simulink model "Leg_Sim_VariableDamping"  (R2020b)
settings: Solver=ode23s  StartTime=0.0  StopTime=1  RelTol=1e-3
values from neighbouring files (symbols this model uses):
  body = Leg_Pars_Body    [Leg_Script_Powered.m]    (also in Leg_Script_Socket_VariableDamping.m; Leg_Script_VariableDamping.m)
  ctrl = Leg_Pars_Ctrl_Powered    [Leg_Script_Powered.m]    (also in Leg_Script_Socket_VariableDamping.m = Leg_Pars_Ctrl_VariableDamping; Leg_Script_VariableDamping.m = Leg_Pars_Ctrl_VariableDamping)
  device = Leg_Pars_Device_Powered    [Leg_Script_Powered.m]    (also in Leg_Script_Socket_VariableDamping.m = Leg_Pars_Device_VariableDamping; Leg_Script_VariableDamping.m = Leg_Pars_Device_VariableDamping)
  FD = [1;1;0;1;1;0;0;1]    [Leg_Script_Powered.m]    (also in Leg_Script_Socket_VariableDamping.m = [1;1;0;1;1;1;1;0;0;1]; Leg_Script_VariableDamping.m)
  human = Leg_Pars_Human(body)    [Leg_Script_Powered.m]    (also in Leg_Script_Socket_VariableDamping.m; Leg_Script_VariableDamping.m)
  intent = [0;1;0]    [Leg_Script_Powered.m]    (also in Leg_Script_Socket_VariableDamping.m; Leg_Script_VariableDamping.m)
  intentv = [1.1;1.1;0.8]    [Leg_Script_Powered.m]    (also in Leg_Script_Socket_VariableDamping.m = [1.1; 1.1; 1.4; 1.4; 1.1; 1.1; 1.4;0.8]; Leg_Script_VariableDamping.m = [1.1; 1.1; 1.4; 1.4; 1.1; 1.1; 1.4;0.8])
  q0 = [0;1;ref.pt_walk ... (first row only)    [Leg_Script_Powered.m]    (also in Leg_Script_Socket_VariableDamping.m; Leg_Script_VariableDamping.m)
  qd0 = [intentv(1)*1.2*intent(1);0;0;0;0;0;0;0]    [Leg_Script_Powered.m]    (also in Leg_Script_Socket_VariableDamping.m = [intentv(1)*1.25*intent(1);0;0;0;0;0;0;0;0;0]; Leg_Script_VariableDamping.m)
  robsim = robotcell2mat(robot)    [Leg_Script_Powered.m]    (also in Leg_Script_Socket_VariableDamping.m; Leg_Script_VariableDamping.m)
  t_intent = [0;1;15]    [Leg_Script_Powered.m]    (also in Leg_Script_Socket_VariableDamping.m = [0;1;35]; Leg_Script_VariableDamping.m = [0;1;35])
  t_intentv = [0;10;15]    [Leg_Script_Powered.m]    (also in Leg_Script_Socket_VariableDamping.m = [0; 9.99; 10; 14.99; 15; 20; 25;35]; Leg_Script_VariableDamping.m = [0; 9.99; 10; 14.99; 15; 20; 25;35])
  u0 = zeros(1,length(robot.gc.body))    [Leg_Script_Powered.m]    (also in Leg_Script_Socket_VariableDamping.m; Leg_Script_VariableDamping.m)
undefined symbols (not defined in the file or in its folder): syst
libraries: simulink x4
(part 2 of 2)

== stateflow chart Leg_Sim_VariableDamping/ctrl/High-level ctrl/Chart ==
  state Walk
    state Swing
      during: tSw = elapsed(sec);
      state SwE
        entry:
        state=5;
      state SwF
        entry:
        state=4;
      (default) -> SwF
      SwF -> SwE [order 1] : [pk<p_5 && wk<-w_0]
    state Stance
      tSt = elapsed(sec);
      tC2PSw = duration(pk<p_3);
      state PSw
        entry:
        state=3;
      state Stand
        state StF
          entry:
          state=1;
        state StE
          entry:
          state=2;
        (default) -> StF
        StF -> StE : [wk<-w_0 && ...
            | duration(pk<p_2)>t_0]
        StE -> StF : [wk>w_1 || ...
            | (wk>w_0 && pk>p_2>t_0)]
      PSw -> Stand [order 2] : [F>F_St ...
          | && pk>p_3 ...
          | && M<M_StX ...
          | || after(t_StX,sec)]
      Stand -> PSw : [M>M_3 && wk>w_0 ...
          | && tC2PSw>t_3]
      (default) -> Stand
    Stance -> Swing : [F<F_Sw ...
        | && pk>p_4]
    SwE -> Stance : [F>F_St ...
        | && pk<p_St ...
        | && after(t_0,sec)]
    SwF -> Stance [order 2] : [F>F_St ...
        | && after(t_0,sec) ...
        | && wk<w_StR && pk<p_StR ...
        | && (pk<p_4 || after(t_StX,sec))]
    PSw -> Swing [order 1] : [F<F_Sw ...
        | || pk>p_4]
    (default) -> Stance
  state InitState
    entry:
    state=0;
  InitState -> Walk : [after(0.1,sec)]
  (default) -> InitState
  data: pk input; wk input; M input; F input; state output; tSw output; tSt output; t_0 constant double =fsm.t_0; p_2 constant double =fsm.p_2; w_1 constant double =fsm.w_1; p_4 constant double =fsm.p_4; p_St constant double =fsm.p_st; w_StR constant double =fsm.w_stR; t_StX constant double =fsm.t_stX; p_StR constant double =fsm.p_stR; M_StX constant double =fsm.M_stX; M_3 constant double =fsm.M_3; t_3 constant double =fsm.t_3; p_3 constant double =fsm.p_3; p_5 constant double =fsm.p_5; w_0 constant double =fsm.w_0; tC2PSw local; F_Sw constant double =fsm.F_Sw; F_St constant double =fsm.F_St

== stateflow chart Leg_Sim_VariableDamping/system/human model/healthy trajectory generator ==
  state Fout = PD2lim(X,Xref,P,D,Flim) [function]
  state Walk
    entry:
    initReStep;
    qcmd(1) = x_heel + l_foot/2;
    qcmd(3) = qs_trunkp_walk;
    during:
    t_ReStep = elapsed(sec);
    t_HeStep = t_ReStep + t_HeStance;
    Ttrunk = PD2lim([q(3) qd(3)],[qref(3) qdref(3)],Ptrr1,Dtrr1,m*5);
    Thip = PD2lim([q(4) qd(4)],[qref(4) qdref(4)],Phip1,Dhip1,m*4);
    state ReStepStart
      during:
      qcmd(4) = interp1x(ts_hip_walkstart, qs_hip_walkstart, t_ReStep/t_ReStep_target);
      state HeSwing
        entry: istate=101;
        F = [0;0];
      state HeStance
        entry: istate=102; initHeStep;
        during:
        t_HeStance = elapsed(sec);
        F = FHeStance;
      Walk.ReStepStart.HeSwing -> Walk.ReStepStart.HeStance : [q(2)<=cos(p_attack)*l_pen_0 ...
          | && after(0.2,sec)]
      (default) -> Walk.ReStepStart.HeSwing
    state ReStepCycle
      during:
      qcmd(4) = interp1x(ts_hip_walk, qs_hip_walk, t_ReStep/t_ReStep_target);
      state DoubleSupport
        entry: istate=110;
        during:
        F = FHeStance;
      state HeSwing
        entry: istate=111;
        F = [0;0];
      state HeStance
        entry: istate=112; initHeStep;
        during:
        t_HeStance = elapsed(sec);
        F = FHeStance;
      Walk.ReStepCycle.HeSwing -> Walk.ReStepCycle.HeStance : [q(2)<=cos(p_attack)*l_pen_0 ...
          | && after(0.2,sec)]
      (default) -> Walk.ReStepCycle.DoubleSupport
      Walk.ReStepCycle.DoubleSupport -> Walk.ReStepCycle.HeSwing : [F_SLIP<0]
    state ReStepStop
      during:
      qcmd(4) = interp1x(ts_hip_stopwalk, qs_hip_stopwalk, t_ReStep/t_ReStep_target);
      state DoubleSupport
        entry: istate=120;
        during:
        F = FHeStance;
      state HeSwing
        entry: istate=121;
        F = [0;0];
      state HeStanceStop
        entry: istate=122; initHeStep;
        during:
        t_HeStance = elapsed(sec);
        F = FHeStance;
      Walk.ReStepStop.HeSwing -> HeStanceStop : [q(2)<=cos(p_attack)*l_pen_0 ...
          | && after(0.2,sec)]
      (default) -> Walk.ReStepStop.DoubleSupport
      Walk.ReStepStop.DoubleSupport -> Walk.ReStepStop.HeSwing : [F_SLIP<0]
  state Init
    entry: qcmd = q0(1:4);
  state Stand
    entry: istate = 0;
    disp(['Stand: t = ' sprintf('%.3f',t) ' s.'])
    t_delay=0.2;
    qcmd = [x_heel+l_foot/2;
    qs_trunky_rest;
    qs_trunkp_rest;
    qs_hip_rest];
    during:
    Ttrunk = PD2lim([q(3) qd(3)],[qref(3) qdref(3)],Ptrr0,Dtrr0,m*2.5);
    Thip = PD2lim([q(4) qd(4)],[qref(4) qdref(4)],Phip0,Dhip0,m*2);
    F = [-50*qd(1);
    m*g*0.5];
  Init -> Walk.ReStepCycle.HeSwing [order 2] : [intent==1]
      | {v_HeAmb_target = intentv;}
  (default) -> Init
  Init -> Stand [order 1] : [intent==0]
  Stand -> ReStepStart : [intent==1]
      | {v_HeAmb_target = intentv;}
  Walk.ReStepStart.HeStance -> (junction 379) : [t_ReStep> t_ReStep_target*0.9 && after(0.2,sec) && fy_heel>1]
  (junction 379) -> ReStepCycle
  (junction 380) -> ReStepCycle [order 1] : [intent==1]
  Walk.ReStepCycle.HeStance -> (junction 380) : [t_ReStep> t_ReStep_target*0.9 && after(0.2,sec) && fy_heel>1]
  HeStanceStop -> Stand : [t_ReStep> t_ReStep_target*0.9 && (qcmd(1)-q(1))<0.01 && after (0.2,sec) && fy_heel>1]
  (junction 380) -> ReStepStop [order 2]
  data: Vq function_output; X function_input; V function_input; Xq function_input; X function_input double size=[1 2]; Xref function_input double size=[1 2]; P function_input double size=1; D function_input double size=1; Fout function_output size=1; Flim function_input double size=1; Fout function_output; qcmd output size=4; fy_heel input; x_heel input; intent input; t_delay output =0.2; ts_hip_walk constant double size=size(ref.th_walk) =ref.th_walk; qs_hip_walk constant double size=size(ref.ph_walk) =ref.ph_walk; qs_trunky_rest constant double =1; qs_trunkp_rest constant double =ref.pt_stand; qs_hip_rest constant double =ref.ph_stand; qs_hip_walkstart constant double size=size(ref.ph_walkstart) =ref.ph_walkstart; ts_hip_walkstart constant double size=size(ref.th_walkstart) =ref.th_walkstart; q0 constant double size=size(q0) =q0; qs_trunkp_walk constant double =ref.pt_walk; istate output =0; l_foot constant double =bdy.x_ball-bdy.x_heel; ts_hip_stopwalk constant double size=size(ref.th_walkstop) =ref.th_walkstop; qs_hip_stopwalk constant double size=size(ref.ph_walkstop) =ref.ph_walkstop; x_Step_est local double =x_step_0; t_ReStep_target local =x_step_0/intentv(1); intentv input; Dtrr1 constant double =imp.Dt_walk; m constant double =bdy.m; q input; qd input; Ptrr1 constant double =imp.Pt_walk; p_attack constant double =SLIP.p_attack; F output; Ttrunk output; Thip output; v_Amb output =intentv(1); Kthrust output =Kthrust_0; F_SLIP local; t_HeStance local =0; Dhip0 constant double =imp.Dh_stand; Phip0 constant double =imp.Ph_stand; Ptrr0 constant double =imp.Pt_stand; g constant double =-rob.gravity(2); Dhip1 constant double =imp.Dh_walk; Phip1 constant double =imp.Ph_walk; q1_Re local =0; m_trunk constant double =bdy.m_trunk; d_slip local; k_slip local; x_pen_0 output; qref input size=4; qdref input size=4; t_HeStep_target local =x_step_0/intentv(1); v_HeAmb_target local =intentv(1); v_HeAmb_target_prev local =intentv(1); v_ReAmb_target local =intentv(1); t_ReStep output =1; v_ReAmb local =intentv(1); v_HeAmb local =intentv(1); q1_He local =0; l_pen_0 local =SLIP.l_rest; Fy_SLIPsupport_max local =0; Dtrr0 constant double =imp.Dt_stand; t input; t_HeStep local =1
  function initReStep:
    | function initReStep
    | disp(['Walk, step residual leg: t = ' sprintf('%.3f',t) ' s.'])
    | % initialize walking parameters
    | % updates
    | q1D = q(1) - q1_Re;
    | q1_Re = q(1);
    | v_ReAmb = q1D/t_ReStep;
    | v_Amb = v_ReAmb;
    | % update time-based targets
    | v_ReAmb_target = intentv;
    | if istate==112
    |     x_Step_est = q1D;
    | end
    | t_ReStep_target = x_Step_est / v_ReAmb_target;
    | t_delay=0.1*t_ReStep_target;
  function Vq = interp1x(X,V,Xq):
    | function Vq = interp1x(X,V,Xq)
    | % interp1x is identical to interp1 except that lower and upper
    | % extrapolation attempts don't result in NaN but in begin and end values,
    | % respectively.
    | Vq = interp1(X,V,max(min(Xq,max(X)),min(X)));
  function initHeStep:
    | function initHeStep
    | disp(['Walk, step intact leg: t = ' sprintf('%.3f',t) ' s.'])
    | % (1) update walking speed
    | q1D = q(1) - q1_He;
    | q1_He = q(1);
    | v_HeAmb = q1D/t_HeStep;
    | v_Amb = v_HeAmb;
    | % set target velocity
    | v_HeAmb_target_prev = v_HeAmb_target; % save previous target
    | v_HeAmb_target = v_ReAmb_target; % new target (= residual leg target velocity)
    | % (2) if not in starting walk stance state, update thrust force
    | if istate ~=102
    |     % use target based on averaging current and previous (simple FIR filter)
    |     v_HeAmb_target_ref = (v_HeAmb_target_prev + v_ReAmb_target)/2;
    |     % calc difference in kinetic energy
    |     ED = m/2*(v_HeAmb_target_ref^2 - v_HeAmb^2);
    |     % adjust thrust force
    |     Kthrust = Kthrust + ED/(x_Step_est*0.5*v_HeAmb_target_ref^2);
    | end
    | % (3)initialize SLIP parameters
    | % calcs
    | t_HeStep_target = x_Step_est / v_HeAmb_target;
    | zeta = 0.2; % damping ratio of SLIP model
    | k_slip = m_trunk*(2*pi/(t_HeStep_target*0.5/2)/sqrt(1-zeta^2))^2;
    | d_slip = zeta*2*sqrt(k_slip*m_trunk); % [Ns/m] damping
    | x_pen_0 = q(1)+sin(p_attack)*l_pen_0;
    | F_SLIP = 0;
    | % SLIP Support
    | Fy_SLIPsupport_max = 0.1*k_slip*(1.1 - v_ReAmb_target);
  function Fout = FHeStance:
    | function Fout = FHeStance
    | % SLIP calculations
    | x_pen = q(1) - x_pen_0;
    | l_pen = sqrt(x_pen^2+q(2)^2);
    | l_pend = (x_pen*qd(1) + q(2)*qd(2))/l_pen;
    | Fk = -k_slip*(l_pen - l_pen_0);
    | Fd = -d_slip*l_pend;
    | F_SLIP = Fk + Fd;
    | Fout = [F_SLIP*x_pen/l_pen;F_SLIP*q(2)/l_pen];
    | 
    | % Add horizontal and vertical support force
    | Fx_support = 0;
    | Fy_support = 0;
    | p_pen = asin(x_pen/l_pen);
    | % Add vertical vertical support force for slow speeds
    | if Fy_SLIPsupport_max>0
    |     p_pen = asin(x_pen/l_pen);
    |     if abs(p_pen)<p_attack
    |         %      Fout(2) = Fout(2) + Fy_SLIPsupport_max/2*(1+cos(p_pen*pi/p_attack));
    |         Fy_support = Fy_SLIPsupport_max*(cos(p_pen*pi/2/p_attack));
    |     end
    | end
    | if istate == 122 % different support for terminating state
    |     % Add horizontal thrust force (without speed change compensation)
    |     Fx_support =  -m*v_HeAmb/(sin(p_attack)*l_pen_0)*qd(1);
    |     % Add addition vertical support for stopping
    |     timefact = max(min(1,1-(t_HeStance-t_HeStep_target/4)/(t_HeStep_target/4)),0);
    |     if abs(p_pen)<p_attack
    |         Fy_support = Fy_support + timefact*0.04*k_slip*(cos(p_pen*pi/2/p_attack));
    |     end
    |     
    | else
    |     % Add horizontal thrust force
    |     Fx_support = v_HeAmb_target^2*Kthrust + ...
    |         0.5*m/2*(v_HeAmb_target^2-v_HeAmb_target_prev^2)/(sin(p_attack)*l_pen_0*2);
    | end
    | 
    | % sum together
    | Fout = Fout + [Fx_support;Fy_support];

== matlab function Leg_Sim_VariableDamping/system/HDgc/HD ==
  data: vJ input; Xup input; v input; Xa input; qdd_id input; tau_fd input; f_ext input; model parameter; fd parameter; qdd_fd output; tau_id output
function [qdd_fd,tau_id] = HD(vJ, Xup, v, Xa, qdd_id, tau_fd, f_ext, model, fd)

% HD  Articulated-Body Hybrid Dynamics Algorithm
% [qdd_fd,tau_id] = HD(vJ, Xup, v, Xa, qdd_id, tau_fd, f_ext, model, fd)
% calculates the hybrid dynamics of a kinematic tree using the articulated-body algorithm. 

% extract statics
ND = model.ND; % 3 = planar, 6 = spatial (note: spatial is not operational in the present implementation)
NB = model.NB;
NB_fd = model.NB_fd;
NB_id = model.NB_id;
S = model.S;
fd_i = model.fd_i;
id_i = model.id_i;
a_grav = model.a_grav;

% pre-allocating variables
c = zeros(ND,NB);
IA = zeros(ND,ND,NB);
pA = zeros(ND,NB);
U = zeros(ND,NB);
d = zeros(NB,1);
u = zeros(NB,1);
a = zeros(ND,NB);

% calculate c (= Sdot*qdot)
for i = 1:NB
    if model.parent(i) ~= 0
        c(:,i) = crm(v(:,i)) * vJ(:,i);
    end
    if fd(i) == 0
        c(:,i) = c(:,i) + S(:,i) * qdd_id(id_i(i));
    end
end

% rigid-body inertia and bias force in body coordinates
for i = 1:NB
    IA(:,:,i) = model.I(:,:,i);
    pA(:,i) = crf(v(:,i)) * model.I(:,:,i) * v(:,i);
    if numel(f_ext)>1 % apply external forces
        pA(:,i) = pA(:,i) - Xa(:,:,i)' \ f_ext(:,i);
    end
end

% forces and inertia [recursive]
for i = NB:-1:1
    if fd(i) == 0
        if model.parent(i) ~= 0
            Ia = IA(:,:,i);
            pa = pA(:,i) + IA(:,:,i)*c(:,i);
            IA(:,:,model.parent(i)) = IA(:,:,model.parent(i)) + Xup(:,:,i)' * Ia * Xup(:,:,i);
            pA(:,model.parent(i)) = pA(:,model.parent(i)) + Xup(:,:,i)' * pa;
        end
    else
        U(:,i) = IA(:,:,i) * S(:,i);
        d(i) = S(:,i)' * U(:,i);
        u(i) = tau_fd(fd_i(i)) - S(:,i)'*pA(:,i);
        if model.parent(i) ~= 0
            Ia = IA(:,:,i) - U(:,i)/d(i)*U(:,i)';
            pa = pA(:,i) + Ia*c(:,i) + U(:,i) * u(i)/d(i);
            IA(:,:,model.parent(i)) = IA(:,:,model.parent(i)) + Xup(:,:,i)' * Ia * Xup(:,:,i);
            pA(:,model.parent(i)) = pA(:,model.parent(i)) + Xup(:,:,i)' * pa;
        end
    end
end

% joint acceleration and torque (in joint space) [recursive]
qdd_fd = zeros(NB_fd,1); 
tau_id = zeros(NB_id,1);

for i = 1:NB
    if model.parent(i) == 0
        a(:,i) = Xup(:,:,i) * -a_grav + c(:,i);
    else
        a(:,i) = Xup(:,:,i) * a(:,model.parent(i)) + c(:,i);
    end
    if fd(i) == 0
        tau_id(id_i(i)) = S(:,i)'*(IA(:,:,i)*a(:,i) + pA(:,i));
    else
        qdd_fd(fd_i(i)) = (u(i) - U(:,i)'*a(:,i))/d(i);
        a(:,i) = a(:,i) + S(:,i)*qdd_fd(fd_i(i));
    end
end

function  vcross = crm( v )

% crm  spatial/planar cross-product operator (motion).
% crm(v)  calculates the 6x6 (or 3x3) matrix such that the expression
% crm(v)*m is the cross product of the motion vectors v and m.  If
% length(v)==6 then it is taken to be a spatial vector, and the return
% value is a 6x6 matrix.  Otherwise, v is taken to be a planar vector, and
% the return value is 3x3.

if length(v) == 6
    
    vcross = [  0    -v(3)  v(2)   0     0     0    ;
        v(3)  0    -v(1)   0     0     0    ;
        -v(2)  v(1)  0      0     0     0    ;
        0    -v(6)  v(5)   0    -v(3)  v(2) ;
        v(6)  0    -v(4)   v(3)  0    -v(1) ;
        -v(5)  v(4)  0     -v(2)  v(1)  0 ];
    
else
    
    vcross = [  0     0     0    ;
        v(3)  0    -v(1) ;
        -v(2)  v(1)  0 ];
end

function  vcross = crf( v )

% crf  spatial/planar cross-product operator (force).
% crf(v)  calculates the 6x6 (or 3x3) matrix such that the expression
% crf(v)*f is the cross product of the motion vector v with the force
% vector f.  If length(v)==6 then it is taken to be a spatial vector, and
% the return value is a 6x6 matrix.  Otherwise, v is taken to be a planar
% vector, and the return value is 3x3.

vcross = -crm(v)';

== matlab function Leg_Sim_VariableDamping/system/HDgc/transcalc ==
  data: q input; qd input; vJ output; model parameter; Xup output; v output; Xa output
function [vJ, Xup, v, Xa] = transcalc( q, qd, model)
% [vJ, Xup, v, Xa] = transcalc( q, qd, model)
% calculates vectors of
% joint velocities vJ;
% body transformations Xup (Xjoint + Xtree);
% body velocities v (w.r.t. global);
% body transformations Xa (w.r.t. global);

% extract statics
ND = model.ND; % 3 = planar, 6 = spatial (note: spatial is not operational in the present implementation)
NB = model.NB;
S = model.S;

% pre-allocating variables
Xup = zeros(ND,ND,NB);
vJ = zeros(ND,NB);

% calculate body transformations and joint velocity
for i = 1:NB
    XJ = jcalc( model.jtype(i,:), q(i) );
    vJ(:,i) = S(:,i)*qd(i);
    Xup(:,:,i) = XJ * model.Xtree(:,:,i);
end

% calculate body velocity and absolute transformations
v = vJ; % 
Xa = Xup; % xform abs coords (pre-allocate)
for i = 1:NB
    if model.parent(i) ~= 0
        v(:,i) = Xup(:,:,i)*v(:,model.parent(i)) + vJ(:,i);
        Xa(:,:,i) = Xup(:,:,i) * Xa(:,:,model.parent(i));
    end
end

function  Xj = jcalc( jtyp, q )

% jcalc  joint transform matrix.
% Xj = jcalc(type,q)  returns the joint transform matrix
% for a joint of the given type.  jtyp can be either a string or a
% structure containing a string-valued field called 'code'.  Either way,
% the string contains the joint type code.  For joints that take
% parameters (e.g. helical), jtyp must be a structure, and it must contain
% a field called 'pars', which in turn is a structure containing one or
% more parameters.  (For a helical joint, pars contains a parameter called
% 'pitch'.)  q is the joint's position variable.

if ischar( jtyp )
    code = jtyp;
else
    code = jtyp.code;
end

switch code % spatial configurations disabled
%     case 'Rx'				% revolute X axis
%         Xj = rotx(q);
%     case 'Ry'				% revolute Y axis
%         Xj = roty(q);
%     case 'Rz'       		% revolute Z axis
%         Xj = rotz(q);
%     case 'Px'				% prismatic X axis
%         Xj = xlt([q 0 0]);
%     case 'Py'				% prismatic Y axis
%         Xj = xlt([0 q 0]);
%     case 'Pz'   			% prismatic Z axis
%         Xj = xlt([0 0 q]);
%     case 'Hz'				% helical (Z axis)
%         Xj = rotz(q) * xlt([0 0 q*jtyp.pars.pitch]);
    case 'rz'				% planar revolute
        Xj = plnr( q, [0 0] );
    case 'px'				% planar prismatic X axis
        Xj = plnr( 0, [q 0] );
    case 'py'				% planar prismatic Y axis
        Xj = plnr( 0, [0 q] );
    otherwise
        error( 'unrecognised joint code ''%s''', code );
end

function  [o1,o2] = plnr( i1, i2 )

% plnr  compose/decompose planar-vector coordinate transform.
% X=plnr(theta,r) and [theta,r]=plnr(X)  compose a planar-vector coordinate
% transform X from its component parts theta and r, and decompose it into
% those parts, respectively.  theta is a scalar and r is a 2D vector.  r is
% returned as a column vector, but it can be supplied as a row or column
% vector.  X is the transform from A to B coordinates, in which frame B is
% located at point r (expressed in A coordinates) and is rotated by an
% angle theta (radians) relative to frame A.  If two arguments are supplied
% then they are assumed to be theta and r, otherwise X.

if nargin == 2				% theta,r --> X
    
    c = cos(i1);
    s = sin(i1);
    
    o1 = [        1          0  0 ;
        s*i2(1)-c*i2(2)   c  s ;
        c*i2(1)+s*i2(2)  -s  c ];
    
else					% X --> theta,r
    
    c = i1(2,2);
    s = i1(2,3);
    
    o1 = atan2(s,c);
    o2 = [ s*i1(2,1)+c*i1(3,1); s*i1(3,1)-c*i1(2,1) ];
    
end

== matlab function Leg_Sim_VariableDamping/system/HDgc/gcPosVel ==
  data: v input; Xa input; xc output; xcd output; model parameter
function [xc,xcd] = gcPosVel( v, Xa, model )

% gcPosVel  calculate positions and velocities of contact points
% [xc,xcd] = gcPosVel(v, Xa,model) calculates 2xn or 3xn matrices,
% depending on whether the model is planar or spatial,
% containing the position xc and linear velocity xcd of every point
% specified in model.gc.point (n==length(model.gc.point)).
% All are expressed in base (i.e., absolute) coordinates.  The
% data for model.gc.point(i) appears in column i.

% pre-allocating variables
ND = model.ND; % 3 = planar, 6 = spatial
xc = zeros(ND/3+1,length(model.gc.body));
xcd = xc;

% calculate contact point position and velocities
for i = 1:model.NB %unique(model.gc.body);
    if any(i==model.gc.body)
    X = inv(Xa(:,:,i));			% xform body i -> abs coords
    va = X * v(:,i);			% body i vel in abs coords
    iset = model.gc.body == i;		% set of points assoc with body i
    pt = Xpt( X, model.gc.point(:,iset), ND );	% xform points to abs coords
    vpt = Vpt( va, pt, ND );			% linear velocities of points
    xc(:,iset) = pt;		% insert into correct columns
    xcd(:,iset) = vpt;
    end
end

function  xp = Xpt( X, p, ND )

% Xpt  apply Plucker/planar coordinate transform to 2D/3D points
% xp=Xpt(X,p,ND)  applies the coordinate transform X to the points in p,
% returning the new coordinates in xp.  If ND==6 then X is taken to be a
% 6x6 matrix and a Plucker coordinate transform, and p is expected to be a
% 3xn matrix of 3D points.  Otherwise, X is assumed to be a planar
% coordinate transform and p a 2xn array of 2D points.

if ND==6			% 3D points
  E = X(1:3,1:3);
  r = -skew(E'*X(4:6,1:3));
else					% 2D points
  E = X(2:3,2:3);
  r = [ X(2,3)*X(2,1)+X(3,3)*X(3,1); X(2,3)*X(3,1)-X(3,3)*X(2,1) ];
end

xp = E * (p - repmat(r(1:2),1,size(p,2)));

function  vp = Vpt( v, p, ND )

% Vpt  spatial/planar velocities --> velocities at points
% vp=Vpt(v,p,ND)  calculates the linear velocities vp at one or more points p
% due to one or more spatial/planar velocities v.  In 3D, v is either 6x1
% or 6xn, and p and vp are 3xn.  In 2D, v is either 3x1 or 3xn, and p and
% vp are 2xn.  If v is just a single spatial/planar vector then it applies
% to every point in p; otherwise, vp(:,i) is calculated from v(:,i) and
% p(:,i).

if size(v,2)==1 && size(p,2)>1
    v_op = repmat(v,1,size(p,2));
else
    v_op = v;
end

if ND==6				% 3D points and velocities
    vp = v_op(4:6,:) + cross(v_op(1:3,:),p,1);
else					% 2D points and velocities
    vp = v_op(2:3,:) + [ -v_op(1,:).*p(2,:); v_op(1,:).*p(1,:) ];
end

% function  out = skew( in )
% 
% % skew  convert 3D vector <--> 3x3 skew-symmetric matrix
% % S=skew(v) and v=skew(A) calculate the 3x3 skew-symmetric matrix S
% % corresponding to the given 3D vector v, and the 3D vector corresponding
% % to the skew-symmetric component of the given arbitrary 3x3 matrix A.  For
% % vectors a and b, skew(a)*b is the cross product of a and b.  If the
% % argument is a 3x3 matrix then it is assumed to be A, otherwise it is
% % assumed to be v.  skew(A) produces a column-vector result, but skew(v)
% % will accept a row or column vector argument.
% 
% if all(size(in)==[3 3])			% do v = skew(A)
%   out = 0.5 * [ in(3,2) - in(2,3);
% 		in(1,3) - in(3,1);
% 		in(2,1) - in(1,2) ];
% else					% do S = skew(v)
%   out = [  0,    -in(3),  in(2);
% 	   in(3),  0,    -in(1);
% 	  -in(2),  in(1),  0 ];
% end

== matlab function Leg_Sim_VariableDamping/system/HDgc/gcontact ==
  data: f output size=[2 length(model.gc.body)]; fcone output size=[1 length(model.gc.body)]; ud output size=[1 length(model.gc.body)]; p input size=[2 length(model.gc.body)]; pd input size=[2 length(model.gc.body)]; u input size=[1 length(model.gc.body)]; model parameter
function [f, fcone, ud] = gcontact( p, pd, u, model)

% gcontact  calculate 2D/3D ground reaction forces due to compliant contact
% [f, fcone, ud] = gcontact(p, pd, u, model)  calculates the ground-reaction
% forces acting on a set of points due to contact with a compliant ground
% plane.  In 3D, the x-y plane is the ground plane, and z is up.  In 2D,
% the x axis is the ground plane and y is up.  
% model.gc.K, model.gc.D and model.gc.mu are scalars
% giving the stiffness, damping and friction coefficients of the ground
% plane.  p and pd are (nD)x(np) matrices giving the positions and
% velocities of a set of np points in nD-dimensional space (nD=2 or 3).
% gcontact uses the size of p to determine whether it is working in 2D or
% 3D space.  u is an (nD-1)x(np) matrix containing the tangential
% deformation state variables used to implement the friction model.  f is
% an (nD)x(np) matrix of calculated ground-reaction forces.  If f(nD,i)==0
% then point i is not in contact; and if f(nD,i)>0 then point i is in
% contact.  ud is the time derivative of u; and fcone is a 1x(np) matrix
% indicating the stick/slip status of each point.  If fcone(i)<=1 then
% point i is sticking.  This can happen only if point i is in contact.

% Implementation note:  This function implements the nonlinear
% spring-damper model described in Azad & Featherstone "Modelling the
% Contact Between a Rolling Sphere and a Compliant Ground Plane", ACRA
% 2010, Brisbane, Australia, Dec. 1-3.  However, the implementation here is
% for points rather than spheres.

% extract relevant parameters from model structure
K = model.gc.K;
D = model.gc.D;
mu = model.gc.mu;

% Normal force calculation
z = p(end,:);
zd = pd(end,:);
zr = sqrt(max(0,-z));

fn = zr .* ((-K)*z - D*zd);

if mu == 0			% special case: modelling frictionless
  f = max( 0, fn );		% contact, so return the normal force now
  return
end

% Algorithm for full normal+tangent force calculation: (1) set all output
% variables to their correct no-contact values; (2) correct all the values
% that are wrong because their respective points are in contact.  Step (2)
% is subdivided into (2a) calculate correct values for sticking; (2b)
% adjust the values for those points that are found to be slipping; (2c)
% make the corrections to the output variables.

% Step 1: set output variables to correct no-contact values

[nd,np] = size(p);
f = zeros(nd,np);
ud = (-K/D) * u;
fcone = repmat(2,1,np);			% 2 is just an arbitrary value > 1

in_ctact = fn > 0;

% Step 2: correct all those values that are wrong because their respective
% points are in contact.  Note: variables with names ending in c have one
% column for each point that is in contact.
if any(in_ctact)

  % Step 2a: calculate correct values for sticking

  fnc = fn(in_ctact);
  udc = pd(1:end-1,in_ctact);

  zrc = repmat(zr(in_ctact),nd-1,1);
  Kc = K * zrc;
  Dc = D * zrc;
  fKc = Kc .* u(:,in_ctact);

  ftc = -fKc - Dc .* udc;		% correct tangent force for sticking

  % now test for slipping

  fslip = mu * fnc;
  if nd == 3				% 3D contact
    ftcmag = sqrt(sum(ftc.^2,1));
  else					% 2D contact
    ftcmag = abs(ftc);
  end
  fconec = ftcmag ./ fslip;
  slipping = fconec > 1;

  % Step 2b: adjust values for those points that are found to be slipping

  if any(slipping)
    attenuator = repmat(fconec(slipping),nd-1,1);
    fts = ftc(:,slipping) ./ attenuator;
    ftc(:,slipping) = fts;
    udc(:,slipping) = -(fts + fKc(:,slipping)) ./ Dc(:,slipping);
  end

  % Step 2c: apply the corrections to the output variables
  
  f(:,in_ctact) = [ftc;fnc];
  ud(:,in_ctact) = udc;
  fcone(in_ctact) = min(2,fconec);

end

== matlab function Leg_Sim_VariableDamping/system/HDgc/Fpt ==
  data: p input; fp input; f_ext output size=[3 model.NB]; model parameter
function  f_ext = Fpt( p, fp , model)

% Fpt  forces at points --> spatial/planar forces
% f_ext = Fpt(p, fp, model)  converts one or more linear forces fp acting
% at one or more points p to their equivalent spatial or planar forces.
% In 3D, fp and p are 3xn arrays and f is 6xn.  In 2D, fp and p are 2xn and
% f is 3xn.  In both cases, f(:,i) is the equivalent of fp(:,i) acting at
% p(:,i).

% extract statics
ND = model.ND; % 3 = planar, 6 = spatial
NB = model.NB;
b = model.gc.body; % b(i) == body number of point i

if ND == 6		% 3D forces at 3D points
  f_gc = [ cross(p,fp,1); fp ];
else					% 2D forces at 2D points
  f_gc = [ p(1,:).*fp(2,:) - p(2,:).*fp(1,:); fp ];
end

% array sizes
f_gc = reshape( f_gc, ND, length(b) );
f_ext = zeros(ND,NB); % pre-allocate
% for each body i that is mentioned at least once, calculate the sum of
% all forces acting on that body
for i = 1:NB
    if any(i==b)
    f_ext(:,i) = sum( f_gc(:,b==i), 2 );
    end
end

== matlab function Leg_Sim_VariableDamping/system/HDgc/Pgc ==
  data: PgcStick output; f input size=[2 length(model.gc.body)]; ud input; pd input; PgcSlip output
function [PgcStick, PgcSlip] = Pgc( f, ud, pd )
% Calculates power loss from sticking (damping) and slipping (sliding).
PgcStick = f(1,:)*ud' + f(2,:)*pd(2,:)';
PgcSlip = f(1,:)*(pd(1,:)-ud)';

== matlab function Leg_Sim_VariableDamping/ctrl/Mid-level ctrl/Mid Ctrl ==
  data: pk input; state input; mid parameter; cmd_m output
function cmd_m = cmds(pk,state,mid)
% pk: knee angle [rad] (old: q)
% state: state {1...5} (integer)
% mid: parameter structure mid-level ctrl

% if nonsense state (e.g. fail, init), make control law act according to:
if all(state~=1:5)
    state = 1;
end

cmd_m = 0;
% % pkd2 = wk_fmed*abs(wk_fmed);
if state==1
    cmd_m = mid.c_StF;
elseif state==2 % velocity max 2 rad/s, torque max 2*75 Nm
    cmd_m = mid.c_StE;
elseif state==3
    cmd_m = mid.c_PSw;
elseif state==4
    cmd_m = mid.c_SwF + mid.c_SwFMax*max(pk-mid.p_SwFMax,0)^2;
elseif state==5
    cmd_m = mid.c_SwE + mid.c_SwEMax*max(mid.p_SwEMax-pk,0)^2;
end

end
